simulink model "ConfigD2"  (R2023a)
settings: Solver=VariableStepAuto  StartTime=0.0  StopTime=370  RelTol=1e-3
values from neighbouring files (symbols this model uses):
  anodeInletPathVolume = 0.03584    [All_Properties.mat]    (also in Valve_Init.m; anode_subsystem_parameters.m)
  molarMassHydrogen = 0.002016    [All_Properties.mat]    (also in Valve_Init.m; anode_subsystem_parameters.m)
  OperatingTemperature = 298    [All_Properties.mat]    (also in Valve_Init.m; anode_subsystem_parameters.m)
  universalGasConstant1 = 8.3145    [All_Properties.mat]    (also in Valve_Init.m; anode_subsystem_parameters.m)
libraries: nesl_utility x17, fl_lib x15, SimscapeFluids_lib x4, slpidlib x1
settings Model: Creator=debjani.ghosh  LastModifiedBy=debjani.ghosh
settings DataIOCC: ReturnWorkspaceOutputs=off
settings SimscapeCC: SimscapeLogType=all  SimscapeLogLimitData=off

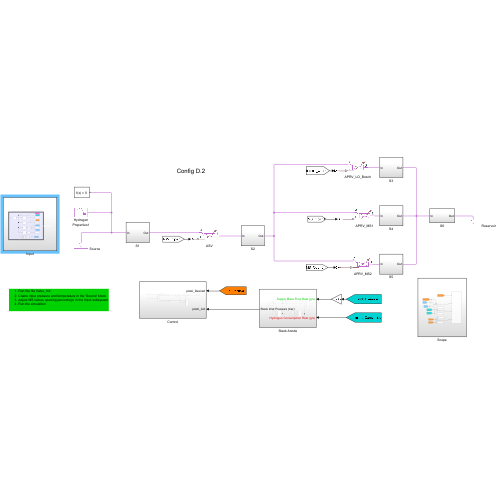
[thumbnail: Simulink's stored preview of the top-level diagram]
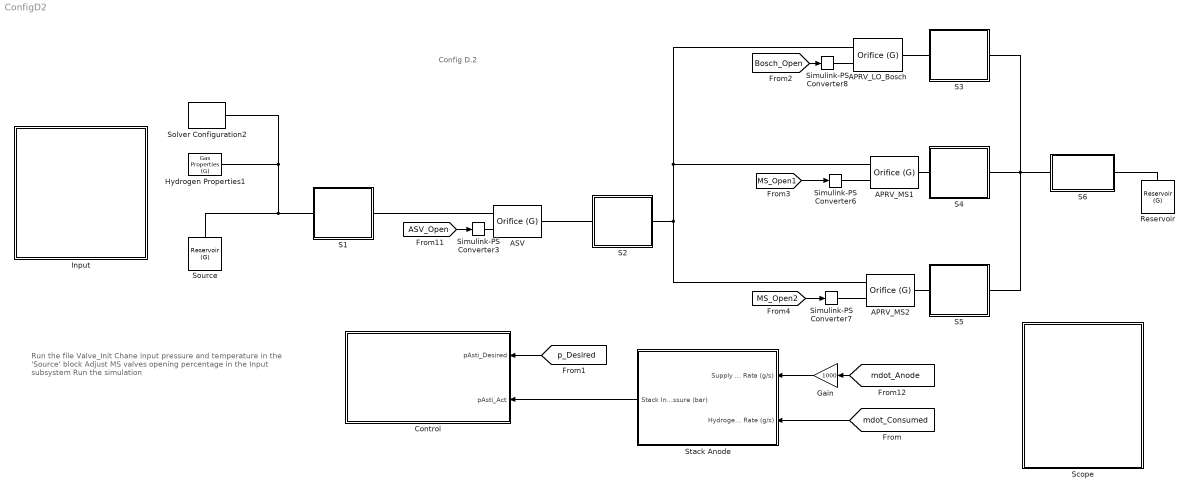
== system ConfigD2 ==
  note: Config D.2
  note: Run the file Valve_Init
      | Chane input pressure and temperature in the 'Source' block
      | Adjust MS valves opening percentage in the Input subsystem
      | Run the simulation
  APRV_LO_Bosch : SimscapeFluids_lib/Gas/Valves & Orifices/Orifice (G)  orifice_type=foundation.enum.constant_variable.variable  orifice_parameterization=fluids.gas.valves_orifices.enum.OrificeParameterization.Cv  opening_characteristic=fluids.gas.valves_orifices.enum.OpeningCharacteristics.Linear  Cv_constant=4  Cv_max=0.15  L_Cv_TLU=0 : 0.2 : 1  Cv_TLU=[1e-06, .8, 1.6, 2.4, 3.2, 4]  xT_Cv=0.6  Kv_constant=3.6  Kv_max=0.32  L_Kv_TLU=0 : 0.2 : 1  Kv_TLU=[1e-06, .72, 1.44, 2.16, 2.88, 3.6]  xT_Kv=0.56  C_constant=12 l/(bar*s)  B_crit_constant=0.3  C_max=12 l/(bar*s)  B_crit_linear=0.3  L_C_TLU=0 : 0.2 : 1  C_TLU=[1e-05, 2.4, 4.8, 7.2, 9.6, 12] l/(bar*s)  B_crit_TLU=0.3 * ones(1, 6)  m=0.5  T_ref_C=293.15 K  rho_ref_C=1.185 kg/m^3  orifice_area_constant=1e-4 m^2  orifice_area_max=5.34e-6 m^2  L_orifice_area_TLU=0 : 0.2 : 1  orifice_area_TLU=[1e-10, 2e-05, 4e-05, 6e-05, 8e-05, .0001] m^2  Cd=0.32  leakage_fraction=1e-6  smoothing_factor=0  B_lam=0.999  area=0.00358 m^2
      settings: LogSimulationData=on  InternalSimscapePortConfiguration="{\"Bottom\":[],\"Left\":[{\"id\":\"A\",\"label\":\"A\",\"type\":\"foundation.gas.gas\"},{\"id\":\"L\",\"label\":\"L\",\"type\":\"input\"}],\"Right\":[{\"id\":\"B\",\"label\":\"B\",\"type\":\"foundation.gas.gas\"}],\"Top\":[]}"
  APRV_MS1 : SimscapeFluids_lib/Gas/Valves & Orifices/Orifice (G)  orifice_type=foundation.enum.constant_variable.variable  orifice_parameterization=fluids.gas.valves_orifices.enum.OrificeParameterization.Kv  opening_characteristic=fluids.gas.valves_orifices.enum.OpeningCharacteristics.Linear  Cv_constant=4  Cv_max=0.24  L_Cv_TLU=0 : 0.2 : 1  Cv_TLU=[1e-06, .8, 1.6, 2.4, 3.2, 4]  xT_Cv=0.7  Kv_constant=3.6  Kv_max=0.32  L_Kv_TLU=0 : 0.2 : 1  Kv_TLU=[1e-06, .72, 1.44, 2.16, 2.88, 3.6]  xT_Kv=0.56  C_constant=12 l/(bar*s)  B_crit_constant=0.3  C_max=12 l/(bar*s)  B_crit_linear=0.3  L_C_TLU=0 : 0.2 : 1  C_TLU=[1e-05, 2.4, 4.8, 7.2, 9.6, 12] l/(bar*s)  B_crit_TLU=0.3 * ones(1, 6)  m=0.5  T_ref_C=293.15 K  rho_ref_C=1.185 kg/m^3  orifice_area_constant=1e-4 m^2  orifice_area_max=5.34e-6 m^2  L_orifice_area_TLU=0 : 0.2 : 1  orifice_area_TLU=[1e-10, 2e-05, 4e-05, 6e-05, 8e-05, .0001] m^2  Cd=0.32  leakage_fraction=1e-6  smoothing_factor=0  B_lam=0.999  area=0.00358 m^2
      settings: LogSimulationData=on  InternalSimscapePortConfiguration="{\"Bottom\":[],\"Left\":[{\"id\":\"A\",\"label\":\"A\",\"type\":\"foundation.gas.gas\"},{\"id\":\"L\",\"label\":\"L\",\"type\":\"input\"}],\"Right\":[{\"id\":\"B\",\"label\":\"B\",\"type\":\"foundation.gas.gas\"}],\"Top\":[]}"
  APRV_MS2 : SimscapeFluids_lib/Gas/Valves & Orifices/Orifice (G)  orifice_type=foundation.enum.constant_variable.variable  orifice_parameterization=fluids.gas.valves_orifices.enum.OrificeParameterization.Kv  opening_characteristic=fluids.gas.valves_orifices.enum.OpeningCharacteristics.Linear  Cv_constant=4  Cv_max=0.24  L_Cv_TLU=0 : 0.2 : 1  Cv_TLU=[1e-06, .8, 1.6, 2.4, 3.2, 4]  xT_Cv=0.7  Kv_constant=3.6  Kv_max=0.32  L_Kv_TLU=0 : 0.2 : 1  Kv_TLU=[1e-06, .72, 1.44, 2.16, 2.88, 3.6]  xT_Kv=0.56  C_constant=12 l/(bar*s)  B_crit_constant=0.3  C_max=12 l/(bar*s)  B_crit_linear=0.3  L_C_TLU=0 : 0.2 : 1  C_TLU=[1e-05, 2.4, 4.8, 7.2, 9.6, 12] l/(bar*s)  B_crit_TLU=0.3 * ones(1, 6)  m=0.5  T_ref_C=293.15 K  rho_ref_C=1.185 kg/m^3  orifice_area_constant=1e-4 m^2  orifice_area_max=5.34e-6 m^2  L_orifice_area_TLU=0 : 0.2 : 1  orifice_area_TLU=[1e-10, 2e-05, 4e-05, 6e-05, 8e-05, .0001] m^2  Cd=0.32  leakage_fraction=1e-6  smoothing_factor=0  B_lam=0.999  area=0.00358 m^2
      settings: LogSimulationData=on  InternalSimscapePortConfiguration="{\"Bottom\":[],\"Left\":[{\"id\":\"A\",\"label\":\"A\",\"type\":\"foundation.gas.gas\"},{\"id\":\"L\",\"label\":\"L\",\"type\":\"input\"}],\"Right\":[{\"id\":\"B\",\"label\":\"B\",\"type\":\"foundation.gas.gas\"}],\"Top\":[]}"
  ASV : SimscapeFluids_lib/Gas/Valves & Orifices/Orifice (G)  orifice_type=foundation.enum.constant_variable.variable  orifice_parameterization=fluids.gas.valves_orifices.enum.OrificeParameterization.Kv  opening_characteristic=fluids.gas.valves_orifices.enum.OpeningCharacteristics.Linear  Cv_constant=4  Cv_max=0.24  L_Cv_TLU=0 : 0.2 : 1  Cv_TLU=[1e-06, .8, 1.6, 2.4, 3.2, 4]  xT_Cv=0.7  Kv_constant=3.6  Kv_max=0.9  L_Kv_TLU=0 : 0.2 : 1  Kv_TLU=[1e-06, .72, 1.44, 2.16, 2.88, 3.6]  xT_Kv=0.56  C_constant=12 l/(bar*s)  B_crit_constant=0.3  C_max=12 l/(bar*s)  B_crit_linear=0.3  L_C_TLU=0 : 0.2 : 1  C_TLU=[1e-05, 2.4, 4.8, 7.2, 9.6, 12] l/(bar*s)  B_crit_TLU=0.3 * ones(1, 6)  m=0.5  T_ref_C=293.15 K  rho_ref_C=1.185 kg/m^3  orifice_area_constant=1e-4 m^2  orifice_area_max=5.34e-6 m^2  L_orifice_area_TLU=0 : 0.2 : 1  orifice_area_TLU=[1e-10, 2e-05, 4e-05, 6e-05, 8e-05, .0001] m^2  Cd=0.32  leakage_fraction=1e-6  smoothing_factor=0  B_lam=0.999  area=0.00358 m^2
      settings: LogSimulationData=on  InternalSimscapePortConfiguration="{\"Bottom\":[],\"Left\":[{\"id\":\"A\",\"label\":\"A\",\"type\":\"foundation.gas.gas\"},{\"id\":\"L\",\"label\":\"L\",\"type\":\"input\"}],\"Right\":[{\"id\":\"B\",\"label\":\"B\",\"type\":\"foundation.gas.gas\"}],\"Top\":[]}"
  Control : Subsystem
  Gain : Gain  Gain=1000
  Hydrogen Properties1 : fl_lib/Gas/Utilities/Gas Properties (G)  gas_spec=foundation.enum.gas_spec.real_gas  R=0.287 kJ/(K*kg)  Z=1  T_ref=293.15 K  h_ref=420 kJ/kg  cp_ref=1 kJ/(K*kg)  mu_ref=18 s*uPa  k_ref=26 mW/(K*m)  T_TLU1=[150 : 10 : 200, 250 : 50 : 1000, 1500, 2000]' K  h_TLU1=[275.264783730547; 285.377054177734; 295.474578903607; 305.560871069627; 315.638490783961; 325.709373787179; 376.008033649461; 426.297784741196; 476.678788323875; 527.253890684429; 578.12722735187; 629.395040865183; 681.137690131207; 733.415442873049; 786.267894376777; 839.715851152006; 893.764459999509; 948.406676876931; 1003.62653219711; 1059.40193232821; 1115.70691941005; 1172.51341226958; 1762.18512007361; 2377.14064127409] kJ/kg  cp_TLU1=[1.01211492398124; 1.01042105529234; 1.00914159006373; 1.00815898273273; 1.00739688341918; 1.00680484569075; 1.00554191216852; 1.00637389921747; 1.0092105862442; 1.01414404435034; 1.02111299587909; 1.02986878923959; 1.04003820504128; 1.05120320041448; 1.06296312852444; 1.07497111709439; 1.08694865668905; 1.0986858495625; 1.11003396604319; 1.12089493621399; 1.13121051694521; 1.14095251451866; 1.21001953144; 1.24628356718428] kJ/(K*kg)  mu_TLU1=[10.3766056544352; 10.9908682444892; 11.5932000841352; 12.1841060353213; 12.764067709023; 13.3335437107148; 16.038149065057; 18.5373404836509; 20.8671495114253; 23.0554226800681; 25.1239717991959; 27.0901379793485; 28.96790749834; 30.7687111230031; 32.5020036481173; 34.17569027566; 35.7964450415303; 37.3699520751368; 38.9010908824946; 40.3940804368247; 41.8525925389218; 43.279841956487; 56.3254722619962; 68.068290080945] s*uPa  k_TLU1=[14.1517155766309; 15.0474512994325; 15.9300520513026; 16.7998749295306; 17.6573089963228; 18.5027588910197; 22.5644026699512; 26.384465676638; 30.0032801168886; 33.4532006033488; 36.7600619429332; 39.9446251241844; 43.0237448740114; 46.0112537033799; 48.9186234516389; 51.7554617696538; 54.5298878921773; 57.2488200454925; 59.9181976996146; 62.5431553064749; 65.128159527924; 67.6771186900213; 91.7815514375552; 114.486299090693] mW/(K*m)  T_TLU2=H2.T K  p_TLU2=H2.p MPa  rho_TLU2=H2.rho kg/m^3  s_TLU2=H2.s kJ/(K*kg)  h_TLU2=H2.h kJ/kg  cp_TLU2=H2.cp kJ/(K*kg)  mu_TLU2=H2.mu s*uPa  k_TLU2=H2.k mW/(K*m)  beta_TLU2=H2.beta MPa  alpha_TLU2=H2.alpha 1/K  T_min_perfect=1 K  T_max_perfect=inf K  p_min_perfect=1 Pa  p_max_perfect=inf MPa  T_range_flag=foundation.enum.T_range_G.from_props  T_min_semiperfect=150 K  T_max_semiperfect=2000 K  p_min_semiperfect=1 Pa  p_max_semiperfect=inf MPa  pT_region_flag=foundation.enum.pT_region_G.from_props  pT_validity_TLU2=ones(24, 20)  T_min_real=150 K  T_max_real=2000 K  p_min_real=0.001 MPa  p_max_real=10 MPa  p_atm=0.101325 MPa  properties_range_check=simscape.enum.assert.action.error  Mach_rev=0.001 / 10
  Input : Subsystem
  Reservoir : fl_lib/Gas/Elements/Reservoir (G)  pressure_spec=foundation.enum.pressure_spec.specified  reservoir_pressure=1.2 bar  reservoir_temperature=298 K  area_A=0.0358 m^2
  S1 : Subsystem
  S2 : Subsystem
  S3 : Subsystem
  S4 : Subsystem
  S5 : Subsystem
  S6 : Subsystem
  Scope : Subsystem
  Simulink-PS Converter{3,6..8} (4 alike) : nesl_utility/Simulink-PS Converter  PhysicalDomain=network_engine_domain  SubClassName=ps_input  LeftPortType=input  RightPortType=output  PseudoPeriodic=off  Frequencies=[]  NoiseDistribution=none  NoiseParameters=[]  Unit=1  AffineConversion=off  FilteringAndDerivatives=provide  SimscapeFilterOrder=1  InputFilterTimeConstant=0.001  UdotUserProvided=0
  Solver Configuration2 : nesl_utility/Solver Configuration  PhysicalDomain=network_engine_domain  SubClassName=solver  LeftPortType=input  RightPortType=generic  Tones=[]  Harmonics=[]  SimulateNoise=off  Profile=off  UseLocalSampling=off  EnableSwitchedLinearOptims=on  FrequencyDomain=off  UseCCode=off  RelTol=0.001  AbsTol=0.001  MinStep=1e-09  ToWorkspace=off  RevertToSquareIcSolve=off  NumHomotopyIterations=100  PhasorMode=off  PhasorModeNumHarmonics=1  ConsistencySolver=NEWTON_XTOL_AFTER_FTOL  IndexReductionMethod=DerivativeReplacement  DoDC=off  ResidualTolerance=1e-09  ConsistencyTolSource=GLOBAL  ConsistencyAbsTol=0.001  ConsistencyRelTol=0.001  ConsistencyTolFactor=0.001  UseLocalSolver=off  LocalSolverChoice=NE_BACKWARD_EULER_ADVANCER  ResolveIndetEquations=on  FunctionEvalNumThread=1  LocalSolverSampleTime=0.001  DoFixedCost=off  MaxNonlinIter=3  MaxModeIter=2  ComputeImpulses=off  ImpulseIterations=2  LinearAlgebra=auto  LinearAlgebraNumThread=0  EquationFormulation=NE_TIME_EF  DelaysMemoryBudget=1024  AutomaticFiltering=on  FilteringTimeConstant=0.001  PartitionStorageMethod=AS_NEEDED  PartitionMemoryBudget=1024  PartitionMethod=ROBUST
  Source : fl_lib/Gas/Elements/Reservoir (G)  pressure_spec=foundation.enum.pressure_spec.specified  reservoir_pressure=12 bar  reservoir_temperature=298 K  area_A=0.0358 m^2
  Stack Anode : Subsystem
  wires:
  [Bosch_Open] -> Simulink-PS Converter8/1
  [MS_Open1] -> Simulink-PS Converter6/1
  [mdot_Consumed] -> Stack Anode/2(Hydrogen Consumption Rate (g/s))
  Gain/1 -> Stack Anode/1(Supply Mass Flow Rate (g/s))
  Stack Anode/1(Stack Inlet Pressure (bar)) -> Control/2(pAsti_Act)
  [p_Desired] -> Control/1(pAsti_Desired)
  [MS_Open2] -> Simulink-PS Converter7/1
  [ASV_Open] -> Simulink-PS Converter3/1
  [mdot_Anode] -> Gain/1
  connections:
  ASV/LConn2 -- Simulink-PS Converter3/RConn1
  S2/LConn1 -- ASV/RConn1
  APRV_MS1/LConn1 -- APRV_MS2/LConn1 -- S2/RConn1 -- APRV_LO_Bosch/LConn1
  S3/RConn1 -- S5/RConn1 -- S6/LConn1 -- S4/RConn1
  APRV_MS2/LConn2 -- Simulink-PS Converter7/RConn1
  APRV_MS1/LConn2 -- Simulink-PS Converter6/RConn1
  APRV_LO_Bosch/LConn2 -- Simulink-PS Converter8/RConn1
  Source/LConn1 -- S1/LConn1 -- Solver Configuration2/RConn1 -- Hydrogen Properties1/RConn1
  S6/RConn1 -- Reservoir/LConn1
  S1/RConn1 -- ASV/LConn1
  S3/LConn1 -- APRV_LO_Bosch/RConn1
  S4/LConn1 -- APRV_MS1/RConn1
  S5/LConn1 -- APRV_MS2/RConn1

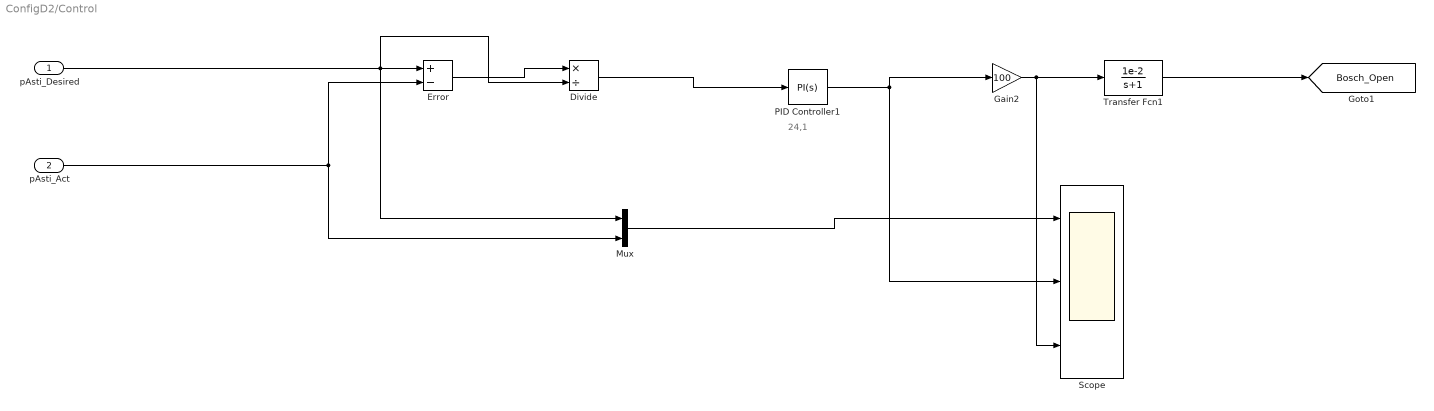
== system ConfigD2/Control ==
  note: 24,1
  pAsti_Desired : Inport
  pAsti_Act : Inport  Port=2
  Divide : Product  Inputs=*/
  Error : Sum  Inputs=+-
  Gain2 : Gain  Gain=100
  Mux : Mux  Inputs=2
  PID Controller1 : slpidlib/PID Controller  Controller=PI  Form=Parallel  TimeDomain=Continuous-time  UseExternalTs=off  SampleTime=-1  IntegratorMethod=Forward Euler  FilterMethod=Forward Euler  ControllerParametersSource=internal  P=20  I=3  UseKiTs=on  D=0.459  N=100  UseFilter=on  TunerSelectOption=Transfer Function Based (PID Tuner App)  InitialConditionSource=internal  InitialConditionForIntegrator=0  InitialConditionForFilter=0  DifferentiatorICPrevScaledInput=0  ExternalReset=none  TrackingMode=off  Kt=1  LimitOutput=on  SatLimitsSource=internal  UpperSaturationLimit=1  LowerSaturationLimit=0  LinearizeAsGain=on  AntiWindupMode=none  Kb=1  LimitIntegrator=off  UpperIntegratorSaturationLimit=inf  LowerIntegratorSaturationLimit=-inf  POutMin=[]  POutMax=[]  IOutMin=[]  IOutMax=[]  DOutMin=[]  DOutMax=[]  NOutMin=[]  NOutMax=[]  SumOutMin=[]  SumOutMax=[]  SaturationOutMin=[]  SaturationOutMax=[]  PParamMin=[]  PParamMax=[]  IParamMin=[]  IParamMax=[]  DParamMin=[]  DParamMax=[]  NParamMin=[]  NParamMax=[]  KbParamMin=[]  KbParamMax=[]  KtParamMin=[]  KtParamMax=[]  KbOutMin=[]  KbOutMax=[]  KtOutMin=[]  KtOutMax=[]  IntegratorOutMin=[]  IntegratorOutMax=[]  FilterOutMin=[]  FilterOutMax=[]  SumI1OutMin=[]  SumI1OutMax=[]  SumI2OutMin=[]  SumI2OutMax=[]  SumI3OutMin=[]  SumI3OutMax=[]  SumI4OutMin=[]  SumI4OutMax=[]  SumDOutMin=[]  SumDOutMax=[]  DifferentiatorOutMin=[]  DifferentiatorOutMax=[]  FilterDiffOutCoefMin=[]  FilterDiffOutCoefMax=[]  ReciprocalOutMin=[]  ReciprocalOutMax=[]  SumDenOutMin=[]  SumDenOutMax=[]  SumNumOutMin=[]  SumNumOutMax=[]  DivideOutMin=[]  DivideOutMax=[]  UdiffTsProdOutMin=[]  UdiffTsProdOutMax=[]  NTsProdOutMin=[]  NTsProdOutMax=[]  UintegralTsProdOutMin=[]  UintegralTsProdOutMax=[]  UngainTsProdOutMin=[]  UngainTsProdOutMax=[]  ClampingZeroOutDataTypeStr=Inherit: Inherit via back propagation  ClampingZeroOutMin=[]  ClampingZeroOutMax=[]  FilterDenConstantOutDataTypeStr=Inherit: Inherit via back propagation  FilterDenConstantOutMin=[]  FilterDenConstantOutMax=[]  PCopyOutDataTypeStr=Inherit: Inherit via back propagation  PCopyOutMin=[]  PCopyOutMax=[]  NCopyOutDataTypeStr=Inherit: Inherit via back propagation  NCopyOutMin=[]  NCopyOutMax=[]  IntegratorContinuousStateAttributes=''  IntegratorStateMustResolveToSignalObject=off  IntegratorRTWStateStorageClass=Auto  FilterContinuousStateAttributes=''  FilterStateMustResolveToSignalObject=off  FilterRTWStateStorageClass=Auto  ParallelPVariant=InternalParameters  IdealPVariant=Disabled  IVariant=InternalParameters  DVariant=Disabled  IntegratorVariant=Continuous  SatVariant=Enabled  AWVariant=Passthrough  PCopyVariant=Disabled  TRVariant=Disabled  FdbkBlocksVariant=Forward  IdealPFdbkVariant=Disabled  SatFdbkVariant=Disabled  DerivativeFilterVariant=Disabled  NVariant=Disabled  NCopyVariant=Disabled_SignalSpec  FilterICVariant=Disabled  IntegratorICVariant=InternalICs  ExternalResetVariant=Disabled  TRSumVariant=Passthrough  SumFdbkVariant=Disabled  SumVariant=Sum_PI  TsampFilterVariant=InternalTs  TsampNgainVariant=Passthrough  TsampIntegralVariant=Disabled_SignalSpec  ExternalSaturationOutDataTypeStr=Inherit: Same as second input
  Scope : Scope  NumInputPorts=3
  Transfer Fcn1 : TransferFcn  Numerator=[1e-2]  Denominator=[1 1]
  tag scope: Bosch_Open=global
  wires:
  Error/1 -> Divide/1
  pAsti_Act/1 -> Mux/2, Error/2
  PID Controller1/1 -> Gain2/1, Scope/2
  Mux/1 -> Scope/1
  pAsti_Desired/1 -> Mux/1, Divide/2, Error/1
  Divide/1 -> PID Controller1/1
  Gain2/1 -> Transfer Fcn1/1, Scope/3
  Transfer Fcn1/1 -> [Bosch_Open]

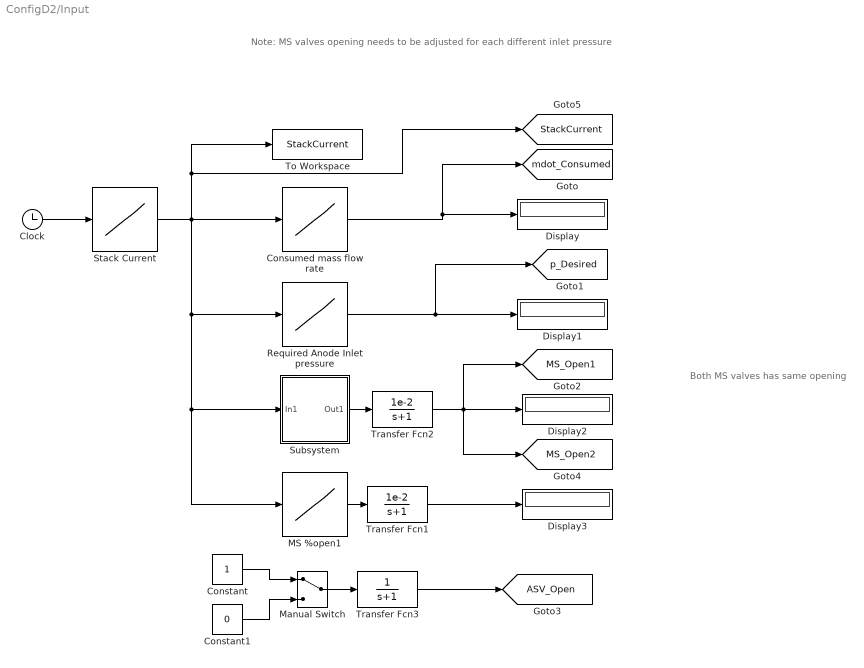
== system ConfigD2/Input ==
  note: Both MS valves has same opening
  note: Note: MS valves opening needs to be adjusted for each different inlet pressure
  Clock : Clock
  Constant : Constant
  Constant1 : Constant  Value=0
  Consumed mass flow rate : Lookup_n-D  NumberOfTableDimensions=1  BreakpointsForDimension1=[0;20;100;200;300;400;500;600]  Table=[0;0.1;0.5;1;1.5;2;2.5;3]  InternalRulePriority=Speed  RndMeth=Simplest
  Display{,1..3} (4 alike) : Display
  MS %open1 : Lookup_n-D  NumberOfTableDimensions=1  BreakpointsForDimension1=[20,100,200,300,400,500,600]  Table=[0;0;0;10;20;30;30]  InternalRulePriority=Speed  RndMeth=Simplest
  Manual Switch : ManualSwitch
  Required Anode Inlet pressure : Lookup_n-D  NumberOfTableDimensions=1  BreakpointsForDimension1=[0;20;100;200;300;400;500;600]  Table=[1;1.4;1.6;1.7;1.8;2;2.3;2.6]  InternalRulePriority=Speed  RndMeth=Simplest
  Stack Current : Lookup_n-D  NumberOfTableDimensions=1  BreakpointsForDimension1=[0;3;5.8;56;58;108;110;160;162;212;214;264;266;316;318;370]  Table=[0;0;20;20;100;100;200;200;300;300;400;400;500;500;600;600]  InternalRulePriority=Speed  RndMeth=Simplest
  Subsystem : Subsystem
  To Workspace : ToWorkspace  VariableName=StackCurrent  SaveFormat=Structure With Time  SampleTime=-1
  Transfer Fcn1 : TransferFcn  Numerator=[1e-2]  Denominator=[1 1]
  Transfer Fcn2 : TransferFcn  Numerator=[1e-2]  Denominator=[1 1]
  Transfer Fcn3 : TransferFcn  Denominator=[1 1]
  tag scope: ASV_Open=global, MS_Open1=global, MS_Open2=global, StackCurrent=global, mdot_Consumed=global, p_Desired=global
  wires:
  Required Anode Inlet pressure/1 -> [p_Desired], Display1/1
  Stack Current/1 -> Subsystem/1(In1), MS %open1/1, Required Anode Inlet pressure/1, To Workspace/1, [StackCurrent], Consumed mass flow rate/1
  MS %open1/1 -> Transfer Fcn1/1
  Consumed mass flow rate/1 -> [mdot_Consumed], Display/1
  Clock/1 -> Stack Current/1
  Transfer Fcn1/1 -> Display3/1
  Transfer Fcn2/1 -> [MS_Open2], [MS_Open1], Display2/1
  Manual Switch/1 -> Transfer Fcn3/1
  Constant1/1 -> Manual Switch/2
  Constant/1 -> Manual Switch/1
  Transfer Fcn3/1 -> [ASV_Open]
  Subsystem/1(Out1) -> Transfer Fcn2/1

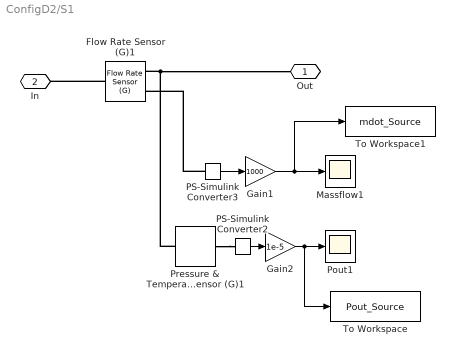
== system ConfigD2/S1 ==
  Flow Rate Sensor (G)1 : fl_lib/Gas/Sensors/Flow Rate Sensor (G)  mass_flow_measure=true  volumetric_flow_measure=false  volumetric_flow_conditions=foundation.enum.volumetric_flow_conditions.actual  p_std=0.101325 MPa  T_std=20 degC  energy_flow_measure=false
      settings: InternalSimscapePortConfiguration="{\"Bottom\":[],\"Left\":[{\"id\":\"A\",\"label\":\"A\",\"type\":\"foundation.gas.gas\"}],\"Right\":[{\"id\":\"B\",\"label\":\"B\",\"type\":\"foundation.gas.gas\"},{\"id\":\"M\",\"label\":\"M\",\"type\":\"output\"}],\"Top\":[]}"
  Gain1 : Gain  Gain=1000
  Gain2 : Gain  Gain=1e-5
  Massflow1 : Scope
  PS-Simulink Converter2 : nesl_utility/PS-Simulink Converter  PhysicalDomain=network_engine_domain  SubClassName=ps_output  LeftPortType=input  RightPortType=output  PseudoPeriodic=off  Frequencies=[]  VectorFormat=inherit  Unit=inherit  AffineConversion=off
  PS-Simulink Converter3 : nesl_utility/PS-Simulink Converter  PhysicalDomain=network_engine_domain  SubClassName=ps_output  LeftPortType=input  RightPortType=output  PseudoPeriodic=off  Frequencies=[]  VectorFormat=inherit  Unit=inherit  AffineConversion=off
  Pout1 : Scope
  Pressure & Temperature Sensor (G)1 : fl_lib/Gas/Sensors/Pressure & Temperature Sensor (G)  reference=foundation.enum.MeasurementReference.absolute  pressure=true  pressure_spec=foundation.enum.PressureMeasementSpec.Absolute  temperature=false
      settings: InternalSimscapePortConfiguration="{\"Bottom\":[],\"Left\":[{\"id\":\"A\",\"label\":\"A\",\"type\":\"foundation.gas.gas\"}],\"Right\":[{\"id\":\"Pa\",\"label\":\"Pa\",\"type\":\"output\"}],\"Top\":[]}"
  To Workspace : ToWorkspace  VariableName=Pout_Source  SaveFormat=Structure With Time  SampleTime=-1
  To Workspace1 : ToWorkspace  VariableName=mdot_Source  SaveFormat=Structure With Time  SampleTime=-1
  Out : PMIOPort  Side=Right
  In : PMIOPort  Port=2  Side=Left
  wires:
  Gain1/1 -> Massflow1/1, To Workspace1/1
  PS-Simulink Converter3/1 -> Gain1/1
  PS-Simulink Converter2/1 -> Gain2/1
  Gain2/1 -> Pout1/1, To Workspace/1
  connections:
  PS-Simulink Converter3/LConn1 -- Flow Rate Sensor (G)1/RConn2
  Flow Rate Sensor (G)1/LConn1 -- In/RConn1
  Pressure & Temperature Sensor (G)1/RConn1 -- PS-Simulink Converter2/LConn1
  Flow Rate Sensor (G)1/RConn1 -- Out/RConn1 -- Pressure & Temperature Sensor (G)1/LConn1

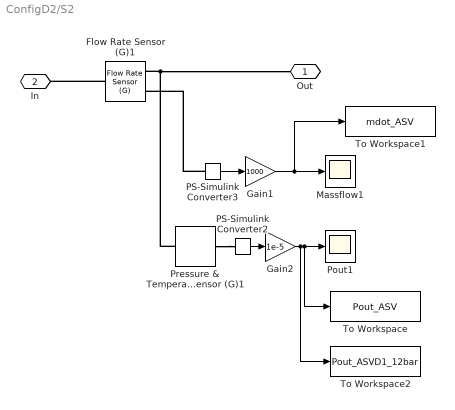
== system ConfigD2/S2 ==
  Flow Rate Sensor (G)1 : fl_lib/Gas/Sensors/Flow Rate Sensor (G)  mass_flow_measure=true  volumetric_flow_measure=false  volumetric_flow_conditions=foundation.enum.volumetric_flow_conditions.actual  p_std=0.101325 MPa  T_std=20 degC  energy_flow_measure=false
      settings: InternalSimscapePortConfiguration="{\"Bottom\":[],\"Left\":[{\"id\":\"A\",\"label\":\"A\",\"type\":\"foundation.gas.gas\"}],\"Right\":[{\"id\":\"B\",\"label\":\"B\",\"type\":\"foundation.gas.gas\"},{\"id\":\"M\",\"label\":\"M\",\"type\":\"output\"}],\"Top\":[]}"
  Gain1 : Gain  Gain=1000
  Gain2 : Gain  Gain=1e-5
  Massflow1 : Scope
  PS-Simulink Converter2 : nesl_utility/PS-Simulink Converter  PhysicalDomain=network_engine_domain  SubClassName=ps_output  LeftPortType=input  RightPortType=output  PseudoPeriodic=off  Frequencies=[]  VectorFormat=inherit  Unit=inherit  AffineConversion=off
  PS-Simulink Converter3 : nesl_utility/PS-Simulink Converter  PhysicalDomain=network_engine_domain  SubClassName=ps_output  LeftPortType=input  RightPortType=output  PseudoPeriodic=off  Frequencies=[]  VectorFormat=inherit  Unit=inherit  AffineConversion=off
  Pout1 : Scope
  Pressure & Temperature Sensor (G)1 : fl_lib/Gas/Sensors/Pressure & Temperature Sensor (G)  reference=foundation.enum.MeasurementReference.absolute  pressure=true  pressure_spec=foundation.enum.PressureMeasementSpec.Absolute  temperature=false
      settings: InternalSimscapePortConfiguration="{\"Bottom\":[],\"Left\":[{\"id\":\"A\",\"label\":\"A\",\"type\":\"foundation.gas.gas\"}],\"Right\":[{\"id\":\"Pa\",\"label\":\"Pa\",\"type\":\"output\"}],\"Top\":[]}"
  To Workspace : ToWorkspace  VariableName=Pout_ASV  SaveFormat=Structure With Time  SampleTime=-1
  To Workspace1 : ToWorkspace  VariableName=mdot_ASV  SaveFormat=Structure With Time  SampleTime=-1
  To Workspace2 : ToWorkspace  VariableName=Pout_ASVD1_12bar  SaveFormat=Structure With Time  SampleTime=-1
  Out : PMIOPort  Side=Right
  In : PMIOPort  Port=2  Side=Left
  wires:
  PS-Simulink Converter2/1 -> Gain2/1
  PS-Simulink Converter3/1 -> Gain1/1
  Gain1/1 -> To Workspace1/1, Massflow1/1
  Gain2/1 -> To Workspace2/1, To Workspace/1, Pout1/1
  connections:
  Pressure & Temperature Sensor (G)1/LConn1 -- Out/RConn1 -- Flow Rate Sensor (G)1/RConn1
  Pressure & Temperature Sensor (G)1/RConn1 -- PS-Simulink Converter2/LConn1
  Flow Rate Sensor (G)1/LConn1 -- In/RConn1
  PS-Simulink Converter3/LConn1 -- Flow Rate Sensor (G)1/RConn2

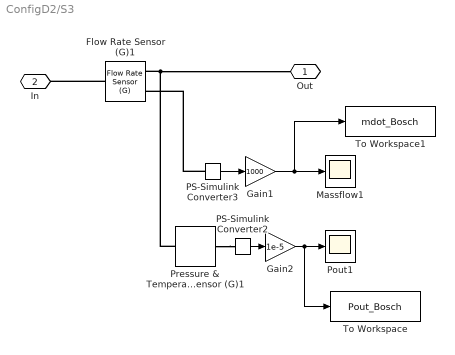
== system ConfigD2/S3 ==
  Flow Rate Sensor (G)1 : fl_lib/Gas/Sensors/Flow Rate Sensor (G)  mass_flow_measure=true  volumetric_flow_measure=false  volumetric_flow_conditions=foundation.enum.volumetric_flow_conditions.actual  p_std=0.101325 MPa  T_std=20 degC  energy_flow_measure=false
      settings: InternalSimscapePortConfiguration="{\"Bottom\":[],\"Left\":[{\"id\":\"A\",\"label\":\"A\",\"type\":\"foundation.gas.gas\"}],\"Right\":[{\"id\":\"B\",\"label\":\"B\",\"type\":\"foundation.gas.gas\"},{\"id\":\"M\",\"label\":\"M\",\"type\":\"output\"}],\"Top\":[]}"
  Gain1 : Gain  Gain=1000
  Gain2 : Gain  Gain=1e-5
  Massflow1 : Scope
  PS-Simulink Converter2 : nesl_utility/PS-Simulink Converter  PhysicalDomain=network_engine_domain  SubClassName=ps_output  LeftPortType=input  RightPortType=output  PseudoPeriodic=off  Frequencies=[]  VectorFormat=inherit  Unit=inherit  AffineConversion=off
  PS-Simulink Converter3 : nesl_utility/PS-Simulink Converter  PhysicalDomain=network_engine_domain  SubClassName=ps_output  LeftPortType=input  RightPortType=output  PseudoPeriodic=off  Frequencies=[]  VectorFormat=inherit  Unit=inherit  AffineConversion=off
  Pout1 : Scope
  Pressure & Temperature Sensor (G)1 : fl_lib/Gas/Sensors/Pressure & Temperature Sensor (G)  reference=foundation.enum.MeasurementReference.absolute  pressure=true  pressure_spec=foundation.enum.PressureMeasementSpec.Absolute  temperature=false
      settings: InternalSimscapePortConfiguration="{\"Bottom\":[],\"Left\":[{\"id\":\"A\",\"label\":\"A\",\"type\":\"foundation.gas.gas\"}],\"Right\":[{\"id\":\"Pa\",\"label\":\"Pa\",\"type\":\"output\"}],\"Top\":[]}"
  To Workspace : ToWorkspace  VariableName=Pout_Bosch  SaveFormat=Structure With Time  SampleTime=-1
  To Workspace1 : ToWorkspace  VariableName=mdot_Bosch  SaveFormat=Structure With Time  SampleTime=-1
  Out : PMIOPort  Side=Right
  In : PMIOPort  Port=2  Side=Left
  wires:
  Gain2/1 -> To Workspace/1, Pout1/1
  PS-Simulink Converter2/1 -> Gain2/1
  PS-Simulink Converter3/1 -> Gain1/1
  Gain1/1 -> To Workspace1/1, Massflow1/1
  connections:
  Pressure & Temperature Sensor (G)1/LConn1 -- Out/RConn1 -- Flow Rate Sensor (G)1/RConn1
  Pressure & Temperature Sensor (G)1/RConn1 -- PS-Simulink Converter2/LConn1
  Flow Rate Sensor (G)1/LConn1 -- In/RConn1
  PS-Simulink Converter3/LConn1 -- Flow Rate Sensor (G)1/RConn2

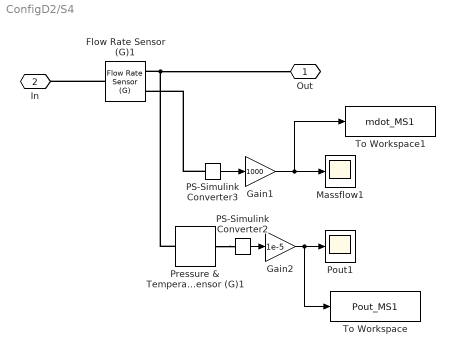
== system ConfigD2/S4 ==
  Flow Rate Sensor (G)1 : fl_lib/Gas/Sensors/Flow Rate Sensor (G)  mass_flow_measure=true  volumetric_flow_measure=false  volumetric_flow_conditions=foundation.enum.volumetric_flow_conditions.actual  p_std=0.101325 MPa  T_std=20 degC  energy_flow_measure=false
      settings: InternalSimscapePortConfiguration="{\"Bottom\":[],\"Left\":[{\"id\":\"A\",\"label\":\"A\",\"type\":\"foundation.gas.gas\"}],\"Right\":[{\"id\":\"B\",\"label\":\"B\",\"type\":\"foundation.gas.gas\"},{\"id\":\"M\",\"label\":\"M\",\"type\":\"output\"}],\"Top\":[]}"
  Gain1 : Gain  Gain=1000
  Gain2 : Gain  Gain=1e-5
  Massflow1 : Scope
  PS-Simulink Converter2 : nesl_utility/PS-Simulink Converter  PhysicalDomain=network_engine_domain  SubClassName=ps_output  LeftPortType=input  RightPortType=output  PseudoPeriodic=off  Frequencies=[]  VectorFormat=inherit  Unit=inherit  AffineConversion=off
  PS-Simulink Converter3 : nesl_utility/PS-Simulink Converter  PhysicalDomain=network_engine_domain  SubClassName=ps_output  LeftPortType=input  RightPortType=output  PseudoPeriodic=off  Frequencies=[]  VectorFormat=inherit  Unit=inherit  AffineConversion=off
  Pout1 : Scope
  Pressure & Temperature Sensor (G)1 : fl_lib/Gas/Sensors/Pressure & Temperature Sensor (G)  reference=foundation.enum.MeasurementReference.absolute  pressure=true  pressure_spec=foundation.enum.PressureMeasementSpec.Absolute  temperature=false
      settings: InternalSimscapePortConfiguration="{\"Bottom\":[],\"Left\":[{\"id\":\"A\",\"label\":\"A\",\"type\":\"foundation.gas.gas\"}],\"Right\":[{\"id\":\"Pa\",\"label\":\"Pa\",\"type\":\"output\"}],\"Top\":[]}"
  To Workspace : ToWorkspace  VariableName=Pout_MS1  SaveFormat=Structure With Time  SampleTime=-1
  To Workspace1 : ToWorkspace  VariableName=mdot_MS1  SaveFormat=Structure With Time  SampleTime=-1
  Out : PMIOPort  Side=Right
  In : PMIOPort  Port=2  Side=Left
  wires:
  Gain1/1 -> Massflow1/1, To Workspace1/1
  PS-Simulink Converter3/1 -> Gain1/1
  PS-Simulink Converter2/1 -> Gain2/1
  Gain2/1 -> Pout1/1, To Workspace/1
  connections:
  PS-Simulink Converter3/LConn1 -- Flow Rate Sensor (G)1/RConn2
  Flow Rate Sensor (G)1/LConn1 -- In/RConn1
  Pressure & Temperature Sensor (G)1/RConn1 -- PS-Simulink Converter2/LConn1
  Flow Rate Sensor (G)1/RConn1 -- Out/RConn1 -- Pressure & Temperature Sensor (G)1/LConn1

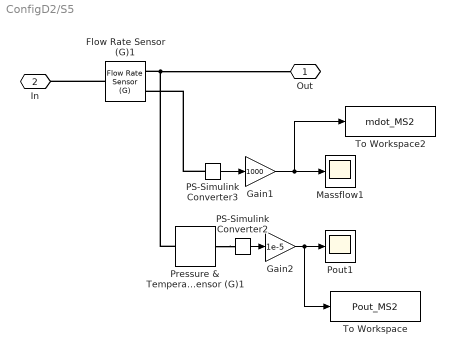
== system ConfigD2/S5 ==
  Flow Rate Sensor (G)1 : fl_lib/Gas/Sensors/Flow Rate Sensor (G)  mass_flow_measure=true  volumetric_flow_measure=false  volumetric_flow_conditions=foundation.enum.volumetric_flow_conditions.actual  p_std=0.101325 MPa  T_std=20 degC  energy_flow_measure=false
      settings: InternalSimscapePortConfiguration="{\"Bottom\":[],\"Left\":[{\"id\":\"A\",\"label\":\"A\",\"type\":\"foundation.gas.gas\"}],\"Right\":[{\"id\":\"B\",\"label\":\"B\",\"type\":\"foundation.gas.gas\"},{\"id\":\"M\",\"label\":\"M\",\"type\":\"output\"}],\"Top\":[]}"
  Gain1 : Gain  Gain=1000
  Gain2 : Gain  Gain=1e-5
  Massflow1 : Scope
  PS-Simulink Converter2 : nesl_utility/PS-Simulink Converter  PhysicalDomain=network_engine_domain  SubClassName=ps_output  LeftPortType=input  RightPortType=output  PseudoPeriodic=off  Frequencies=[]  VectorFormat=inherit  Unit=inherit  AffineConversion=off
  PS-Simulink Converter3 : nesl_utility/PS-Simulink Converter  PhysicalDomain=network_engine_domain  SubClassName=ps_output  LeftPortType=input  RightPortType=output  PseudoPeriodic=off  Frequencies=[]  VectorFormat=inherit  Unit=inherit  AffineConversion=off
  Pout1 : Scope
  Pressure & Temperature Sensor (G)1 : fl_lib/Gas/Sensors/Pressure & Temperature Sensor (G)  reference=foundation.enum.MeasurementReference.absolute  pressure=true  pressure_spec=foundation.enum.PressureMeasementSpec.Absolute  temperature=false
      settings: InternalSimscapePortConfiguration="{\"Bottom\":[],\"Left\":[{\"id\":\"A\",\"label\":\"A\",\"type\":\"foundation.gas.gas\"}],\"Right\":[{\"id\":\"Pa\",\"label\":\"Pa\",\"type\":\"output\"}],\"Top\":[]}"
  To Workspace : ToWorkspace  VariableName=Pout_MS2  SaveFormat=Structure With Time  SampleTime=-1
  To Workspace2 : ToWorkspace  VariableName=mdot_MS2  SaveFormat=Structure With Time  SampleTime=-1
  Out : PMIOPort  Side=Right
  In : PMIOPort  Port=2  Side=Left
  wires:
  Gain2/1 -> To Workspace/1, Pout1/1
  PS-Simulink Converter2/1 -> Gain2/1
  PS-Simulink Converter3/1 -> Gain1/1
  Gain1/1 -> To Workspace2/1, Massflow1/1
  connections:
  Pressure & Temperature Sensor (G)1/LConn1 -- Out/RConn1 -- Flow Rate Sensor (G)1/RConn1
  Pressure & Temperature Sensor (G)1/RConn1 -- PS-Simulink Converter2/LConn1
  Flow Rate Sensor (G)1/LConn1 -- In/RConn1
  PS-Simulink Converter3/LConn1 -- Flow Rate Sensor (G)1/RConn2

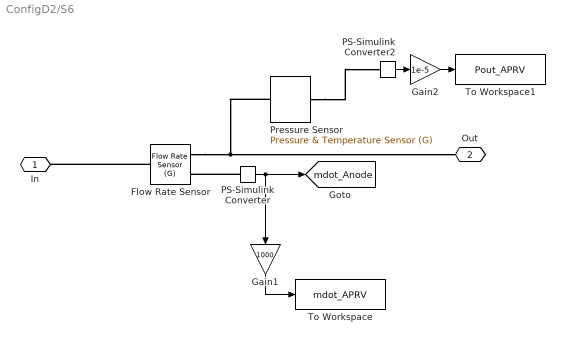
== system ConfigD2/S6 ==
  Flow Rate Sensor : fl_lib/Gas/Sensors/Flow Rate Sensor (G)  mass_flow_measure=true  volumetric_flow_measure=false  volumetric_flow_conditions=foundation.enum.volumetric_flow_conditions.actual  p_std=0.101325 MPa  T_std=20 degC  energy_flow_measure=false
      settings: InternalSimscapePortConfiguration="{\"Bottom\":[],\"Left\":[{\"id\":\"A\",\"label\":\"A\",\"type\":\"foundation.gas.gas\"}],\"Right\":[{\"id\":\"B\",\"label\":\"B\",\"type\":\"foundation.gas.gas\"},{\"id\":\"M\",\"label\":\"M\",\"type\":\"output\"}],\"Top\":[]}"
  Gain1 : Gain  Gain=1000
  Gain2 : Gain  Gain=1e-5
  PS-Simulink Converter : nesl_utility/PS-Simulink Converter  PhysicalDomain=network_engine_domain  SubClassName=ps_output  LeftPortType=input  RightPortType=output  PseudoPeriodic=off  Frequencies=[]  VectorFormat=inherit  Unit=inherit  AffineConversion=off
  PS-Simulink Converter2 : nesl_utility/PS-Simulink Converter  PhysicalDomain=network_engine_domain  SubClassName=ps_output  LeftPortType=input  RightPortType=output  PseudoPeriodic=off  Frequencies=[]  VectorFormat=inherit  Unit=inherit  AffineConversion=off
  "Pressure Sensor " : fl_lib/Gas/Sensors/Pressure & Temperature Sensor (G)  reference=foundation.enum.MeasurementReference.absolute  pressure=true  pressure_spec=foundation.enum.PressureMeasementSpec.Absolute  temperature=false
      settings: InternalSimscapePortConfiguration="{\"Bottom\":[],\"Left\":[{\"id\":\"A\",\"label\":\"A\",\"type\":\"foundation.gas.gas\"}],\"Right\":[{\"id\":\"Pa\",\"label\":\"Pa\",\"type\":\"output\"}],\"Top\":[]}"
  To Workspace : ToWorkspace  VariableName=mdot_APRV  SaveFormat=Structure With Time  SampleTime=-1
  To Workspace1 : ToWorkspace  VariableName=Pout_APRV  SaveFormat=Structure With Time  SampleTime=-1
  In : PMIOPort  Side=Left
  Out : PMIOPort  Port=2  Side=Right
  tag scope: mdot_Anode=global
  wires:
  PS-Simulink Converter/1 -> [mdot_Anode], Gain1/1
  PS-Simulink Converter2/1 -> Gain2/1
  Gain2/1 -> To Workspace1/1
  Gain1/1 -> To Workspace/1
  connections:
  "Pressure Sensor "/LConn1 -- Out/RConn1 -- Flow Rate Sensor/RConn1
  PS-Simulink Converter/LConn1 -- Flow Rate Sensor/RConn2
  Flow Rate Sensor/LConn1 -- In/RConn1
  "Pressure Sensor "/RConn1 -- PS-Simulink Converter2/LConn1

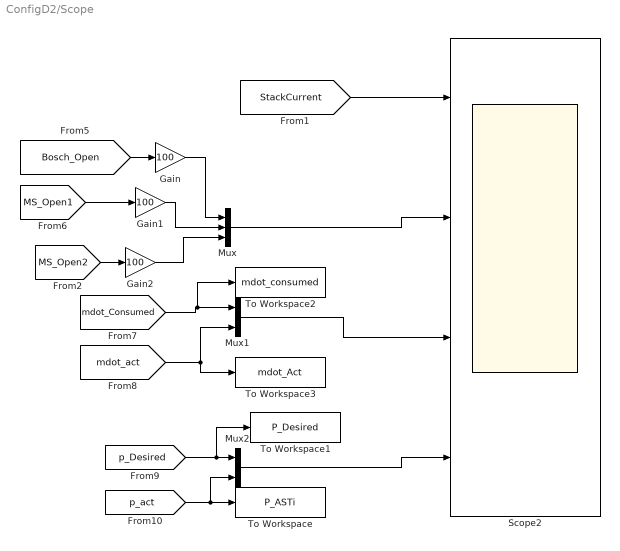
== system ConfigD2/Scope ==
  Gain : Gain  Gain=100
  Gain1 : Gain  Gain=100
  Gain2 : Gain  Gain=100
  Mux : Mux  Inputs=3
  Mux1 : Mux  Inputs=2
  Mux2 : Mux  Inputs=2
  Scope2 : Scope  NumInputPorts=4
  To Workspace : ToWorkspace  VariableName=P_ASTi  SaveFormat=Structure With Time  SampleTime=-1
  To Workspace1 : ToWorkspace  VariableName=P_Desired  SaveFormat=Structure With Time  SampleTime=-1
  To Workspace2 : ToWorkspace  VariableName=mdot_consumed  SaveFormat=Structure With Time  SampleTime=-1
  To Workspace3 : ToWorkspace  VariableName=mdot_Act  SaveFormat=Structure With Time  SampleTime=-1
  wires:
  [p_Desired] -> To Workspace1/1, Mux2/1
  Mux/1 -> Scope2/2
  Mux1/1 -> Scope2/3
  [mdot_act] -> To Workspace3/1, Mux1/2
  Mux2/1 -> Scope2/4
  [Bosch_Open] -> Gain/1
  [p_act] -> Mux2/2, To Workspace/1
  [mdot_Consumed] -> To Workspace2/1, Mux1/1
  [MS_Open1] -> Gain1/1
  [StackCurrent] -> Scope2/1
  [MS_Open2] -> Gain2/1
  Gain/1 -> Mux/1
  Gain1/1 -> Mux/2
  Gain2/1 -> Mux/3

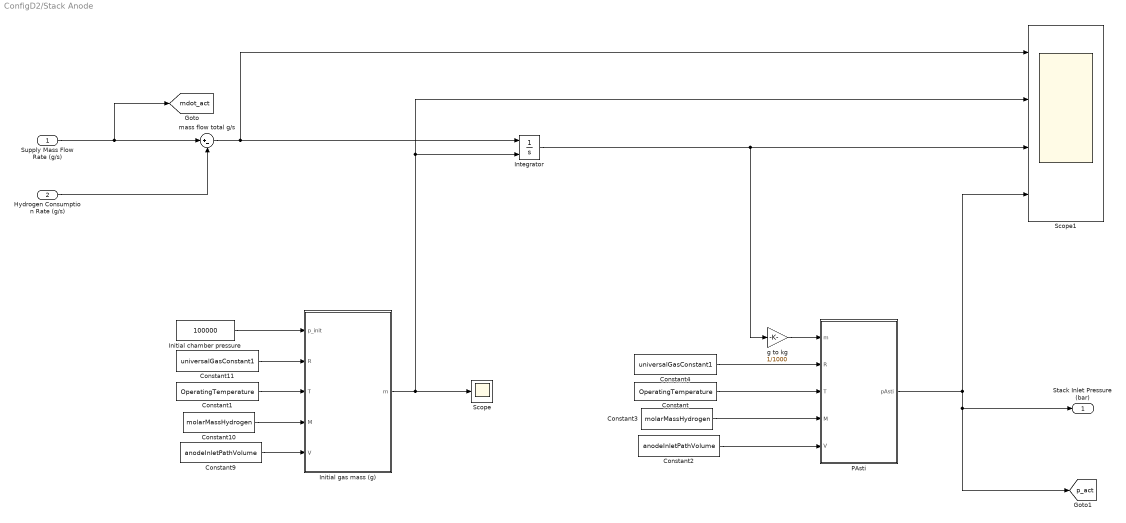
== system ConfigD2/Stack Anode ==
  Supply Mass Flow Rate (g/s) : Inport
  Hydrogen Consumption Rate (g/s) : Inport  Port=2
  Constant : Constant  Value=OperatingTemperature
  Constant1 : Constant  Value=OperatingTemperature
  Constant10 : Constant  Value=molarMassHydrogen
  Constant11 : Constant  Value=universalGasConstant1
  Constant2 : Constant  Value=anodeInletPathVolume
  Constant3 : Constant  Value=molarMassHydrogen
  Constant4 : Constant  Value=universalGasConstant1
  Constant9 : Constant  Value=anodeInletPathVolume
  Initial chamber pressure : Constant  Value=100000
  Initial gas mass (g) : MATLAB Function  TreatAsAtomicUnit=on
  Integrator : Integrator  InitialConditionSource=external
  PAsti : MATLAB Function  TreatAsAtomicUnit=on
  Scope : Scope
  Scope1 : Scope  NumInputPorts=4
  g to kg : Gain  Gain=1/1000
  mass flow total g/s : Sum  Inputs=|+-
  Stack Inlet Pressure (bar) : Outport
  tag scope: mdot_act=global, p_act=global
  wires:
  Initial chamber pressure/1 -> Initial gas mass (g)/1(p_init)
  Constant/1 -> PAsti/3(T)
  Constant4/1 -> PAsti/2(R)
  Constant3/1 -> PAsti/4(M)
  Constant2/1 -> PAsti/5(V)
  Constant11/1 -> Initial gas mass (g)/2(R)
  Constant1/1 -> Initial gas mass (g)/3(T)
  Constant10/1 -> Initial gas mass (g)/4(M)
  Constant9/1 -> Initial gas mass (g)/5(V)
  mass flow total g/s/1 -> Integrator/1, Scope1/1
  Hydrogen Consumption Rate (g/s)/1 -> mass flow total g/s/2
  Supply Mass Flow Rate (g/s)/1 -> [mdot_act], mass flow total g/s/1
  g to kg/1 -> PAsti/1(m)
  Initial gas mass (g)/1(m) -> Scope1/2, Integrator/2, Scope/1
  Integrator/1 -> g to kg/1, Scope1/3
  PAsti/1(pAsti) -> Scope1/4, Stack Inlet Pressure (bar)/1, [p_act]

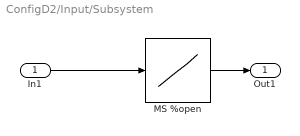
== system ConfigD2/Input/Subsystem ==
  In1 : Inport
  MS %open : Lookup_n-D  NumberOfTableDimensions=1  BreakpointsForDimension1=[20,100,200,300,400,500,600]  Table=[0;0;0;0;10;20;30]  InternalRulePriority=Speed  RndMeth=Simplest
  Out1 : Outport
  wires:
  MS %open/1 -> Out1/1
  In1/1 -> MS %open/1

== matlab function ConfigD2/Stack Anode/Initial gas mass (g) ==
  data: p_init input; m output; R input; T input; M input; V input
function m = fcn(p_init,R,T,M,V)

%from Ideal Gas Law

m = 1000*((p_init * M * V) / (R * T));  %mass in g

== matlab function ConfigD2/Stack Anode/PAsti ==
  data: m input; pAsti output; R input; T input; M input; V input
function pAsti = fcn(m,R,T,M,V)

%from Ideal Gas Law

p = (m * R * T) / (M * V);  %Pressure in Pa

pAsti =p * 1e-5;  % Pressure in bar
